simulink model "ShearFrameStru_3F_sinInput"  (R2016b)
settings: Solver=ode5  StartTime=0.0  StopTime=Tsim  FixedStep=dt  RelTol=1e-3
values from neighbouring files (symbols this model uses):
  A1 = 1/(beta*dt^2)    [Newmark_dsmj.m]    (also in SFstru_sinInput.m = 1)
  A2 = gama/(beta*dt)    [Newmark_dsmj.m]    (also in SFstru_sinInput.m = 1)
  A3 = 1/(beta*dt)    [Newmark_dsmj.m]    (also in SFstru_sinInput.m = 1)
  Abw = [zeros(DoF) ,   eye(DoF) ... (first row only)    [SFstru_sinInput.m]
  Bbw = [zeros(DoF,2*DoF) ... (first row only)    [SFstru_sinInput.m]
  Cbw = [temp_matrix,zeros(DoF) ... (first row only)    [SFstru_sinInput.m]
  Dbw = zeros(2*DoF,2*DoF)    [SFstru_sinInput.m]
  gamma1 = yita1    (= 4882812.5)    [SFstru_sinInput.m]
  gamma2 = yita2    (= 4882812.5)    [SFstru_sinInput.m]
  gamma3 = yita3    (= 4882812.5)    [SFstru_sinInput.m]
  n1 = 5    [SFstru_sinInput.m]
  n2 = 5    [SFstru_sinInput.m]
  n3 = 5    [SFstru_sinInput.m]
  yita1 = 1/(2*uy1^n1)    (= 4882812.5)    [SFstru_sinInput.m]
  yita2 = 1/(2*uy2^n2)    (= 4882812.5)    [SFstru_sinInput.m]
  yita3 = 1/(2*uy3^n3)    (= 4882812.5)    [SFstru_sinInput.m]
settings Model: Creator=dsmj  LastModifiedBy=Maijia Su

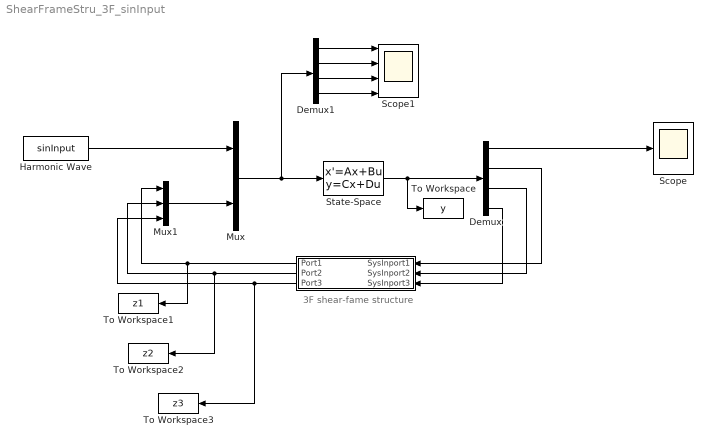
== system ShearFrameStru_3F_sinInput ==
  note: 3F shear-fame structure
  " " : Subsystem  mask(Differential Equation Editor (DEE)){}
      settings: OpenFcn=diffeqed
      mask Display: disp('Bouc-Wen model')
  Demux : Demux  Outputs=[3,1,1,1]
  Demux1 : Demux
  Harmonic Wave : FromWorkspace  VariableName=sinInput  SampleTime=0
  Mux : Mux  Inputs=2
  Mux1 : Mux  Inputs=3
  Scope : Scope
  Scope1 : Scope  NumInputPorts=4
  State-Space : StateSpace  A=Abw  B=Bbw  C=Cbw  D=Dbw  X0=0
  To Workspace : ToWorkspace  VariableName=y  SaveFormat=Timeseries  SampleTime=-1
  To Workspace1 : ToWorkspace  VariableName=z1  SaveFormat=Timeseries  SampleTime=-1
  To Workspace2 : ToWorkspace  VariableName=z2  SaveFormat=Timeseries  SampleTime=-1
  To Workspace3 : ToWorkspace  VariableName=z3  SaveFormat=Timeseries  SampleTime=-1
  wires:
  State-Space/1 -> To Workspace/1, Demux/1
  Mux/1 -> Demux1/1, State-Space/1
  " "/1(Port1) -> To Workspace1/1, Mux1/1
  Mux1/1 -> Mux/2
  Demux1/1 -> Scope1/1
  Demux1/2 -> Scope1/2
  Demux1/3 -> Scope1/3
  " "/2(Port2) -> To Workspace2/1, Mux1/2
  Demux/2 -> " "/1(SysInport1)
  Demux/4 -> " "/3(SysInport3)
  Demux/3 -> " "/2(SysInport2)
  " "/3(Port3) -> To Workspace3/1, Mux1/3
  Demux1/4 -> Scope1/4
  Harmonic Wave/1 -> Mux/1
  Demux/1 -> Scope/1

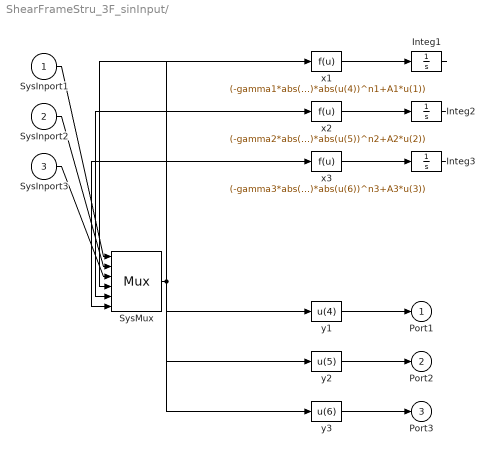
== system ShearFrameStru_3F_sinInput/  ==
  SysInport1 : Inport
  SysInport2 : Inport  Port=2
  SysInport3 : Inport  Port=3
  Integ1 : Integrator
  Integ2 : Integrator
  Integ3 : Integrator
  SysMux : Mux  Inputs=6
  x1 : Fcn  Expr=(-gamma1*abs(u(1))*abs(u(4))^(n1-1)*u(4)-yita1*u(1)*abs(u(4))^n1+A1*u(1))
  x2 : Fcn  Expr=(-gamma2*abs(u(2))*abs(u(5))^(n2-1)*u(5)-yita2*u(2)*abs(u(5))^n2+A2*u(2))
  x3 : Fcn  Expr=(-gamma3*abs(u(3))*abs(u(6))^(n3-1)*u(6)-yita3*u(3)*abs(u(6))^n3+A3*u(3))
  y1 : Fcn  Expr=u(4)
  y2 : Fcn  Expr=u(5)
  y3 : Fcn  Expr=u(6)
  Port1 : Outport
  Port2 : Outport  Port=2
  Port3 : Outport  Port=3
  wires:
  SysInport1/1 -> SysMux/1
  SysInport2/1 -> SysMux/2
  SysInport3/1 -> SysMux/3
  SysMux/1 -> x1/1, x2/1, x3/1, y1/1, y2/1, y3/1
  x1/1 -> Integ1/1
  Integ1/1 -> SysMux/4
  x2/1 -> Integ2/1
  Integ2/1 -> SysMux/5
  x3/1 -> Integ3/1
  Integ3/1 -> SysMux/6
  y1/1 -> Port1/1
  y2/1 -> Port2/1
  y3/1 -> Port3/1
